simulink model "Disturbed_H_PB"  (R2023a)
settings: Solver=VariableStepAuto  StartTime=0.0  StopTime=ttot  RelTol=1e-3
InitFcn:
  | run("Trajectory_Planning_Francesco.m");
  | 
  | % Defining important terms
  | 
  | g=9.81;
  | A=[zeros(3) eye(3);zeros(3) zeros(3)];
  | B=[zeros(3);eye(3)];
  | 
  | % Computing gain PD+
  | 
  | Ke_He=[diag([10 10 10]),diag([10 10 10])];
  | Kp_He=[diag([100 100 100]),diag([1 1 10])];
  | 
  | Kp_PB=[100*diag([1 1 1]),diag([0.5 0.5 10])];
values from neighbouring files (symbols this model uses):
  Ib = diag([1.2416 1.2416 2*1.2416])    [Trajectory_Planning_Francesco.m]
  K3 = flip(G3.Denominator{1})    [Trajectory_Planning_Francesco.m]
  lin_vel_0 = [dot_x0 dot_y0 dot_z0]    [Trajectory_Planning_Francesco.m]
  mass = 1.2    [Trajectory_Planning_Francesco.m]
  pos_0 = [Poses(1,1) Poses(1,2) Poses(1,3)]    [Trajectory_Planning_Francesco.m]
  Ts = 0.001    [Trajectory_Planning_Francesco.m]
undefined symbols (not defined in the file or in its folder): DiscIntNeverNeededParam
libraries: robotcorelib x2, uavutilslib x2
settings Model: Creator=fabioruggiero  LastModifiedBy=39388
settings ModelReferenceCC: EnableRefExpFcnMdlSchedulingChecks=on

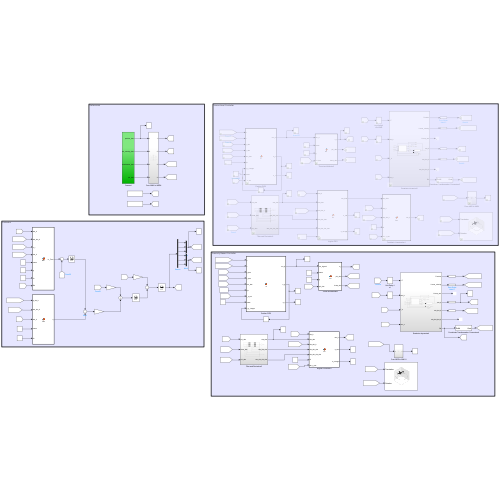
[thumbnail: Simulink's stored preview of the top-level diagram]
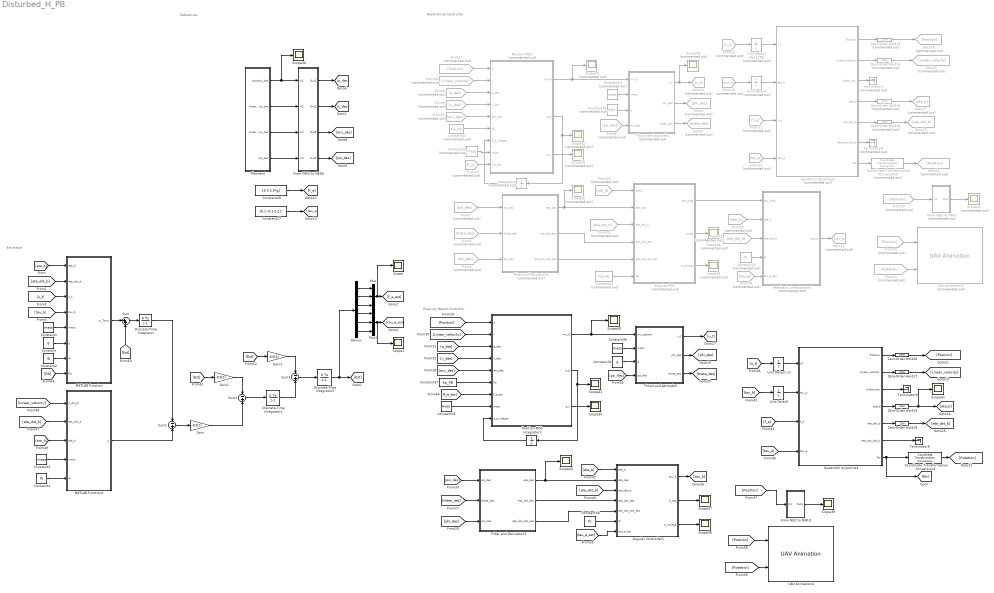
== system Disturbed_H_PB ==
  note: Estimator
  note: References
  note: Hierarchical Controller
  note: Passivity Based Controller
  Angular Controller1 : MATLAB Function  TreatAsAtomicUnit=on
  Angular PID1 : MATLAB Function  Commented=on  TreatAsAtomicUnit=on
  Constant : Constant  Value=g
  Constant{1,3,35..36} (4 alike) : Constant  Value=mass
  Constant18 : Constant  Commented=on  Value=9.81
  Constant19 : Constant  Commented=on  Value=Ib
  Constant2 : Constant  Value=Ib
  Constant20 : Constant  Commented=on  Value=mass
  Constant21 : Constant  Commented=on  Value=Kp_He
  Constant22 : Constant  Commented=on  Value=Ke_He
  Constant23 : Constant  Commented=on  Value=mass
  Constant27 : Constant  Value=[0.1 -0.1 0.2]'  SampleTime=Ts
  Constant28 : Constant  Value=[0 0 2.5*g]  SampleTime=Ts
  Constant34 : Constant  Value=g
  Constant37 : Constant  Value=Kp_PB
  Constant38 : Constant  Value=Ib
  Constant4 : Constant  Value=Ib
  Coordinate Transformation Conversion3 : robotcorelib/Coordinate Transformation Conversion  Commented=on  InputRepresentation=Rotation Matrix  InputEulerSequence=ZYX  ShowTrVecInputPort=on  OutputRepresentation=Quaternion  OutputEulerSequence=ZYX  ShowTrVecOutputPort=on  SimulateUsing=Interpreted execution
  Coordinate Transformation Conversion4 : robotcorelib/Coordinate Transformation Conversion  InputRepresentation=Rotation Matrix  InputEulerSequence=ZYX  ShowTrVecInputPort=on  OutputRepresentation=Quaternion  OutputEulerSequence=ZYX  ShowTrVecOutputPort=on  SimulateUsing=Interpreted execution
  Demux : Demux  Outputs=6
  Discrete-Time Integrator : DiscreteIntegrator  gainval=1  SampleTime=Ts  ICPrevOutput=DiscIntNeverNeededParam  ICPrevScaledInput=DiscIntNeverNeededParam
  Discrete-Time Integrator1 : DiscreteIntegrator  gainval=1  SampleTime=Ts  ICPrevOutput=DiscIntNeverNeededParam  ICPrevScaledInput=DiscIntNeverNeededParam
  Discrete-Time Integrator2 : DiscreteIntegrator  gainval=1  SampleTime=Ts  ICPrevOutput=DiscIntNeverNeededParam  ICPrevScaledInput=DiscIntNeverNeededParam
  Feedback Linearization1 : MATLAB Function  Commented=on  TreatAsAtomicUnit=on
  Filter and Derivation2 : Subsystem  Commented=on
  Filter and Derivation3 : Subsystem
  From NED to NWU : Subsystem  Commented=on
  From NED to NWU1 : Subsystem
  From NWU to NED6 : Subsystem
  From10 : From  Commented=on  GotoTag=acc_des
  From11 : From  Commented=on  GotoTag=f_e
  From12 : From  Commented=on  GotoTag=tau_e
  From13 : From  Commented=on  GotoTag=f_e
  From14 : From  Commented=on  GotoTag=tau_e
  From15 : From  Commented=on  GotoTag=u_t
  From16 : From  Commented=on  GotoTag=tau_b
  From17 : From  Commented=on  GotoTag=Position
  From18 : From  Commented=on  GotoTag=Linear_velocity
  From19 : From  Commented=on  GotoTag=Position
  From20 : From  Commented=on  GotoTag=Position
  From21 : From  Commented=on  GotoTag=Rotation
  From22 : From  Commented=on  GotoTag=eta_b
  From23 : From  Commented=on  GotoTag=eta_b
  From24 : From  Commented=on  GotoTag=eta_dot_b
  From25 : From  Commented=on  GotoTag=eta_dot_b
  From4 : From  Commented=on  GotoTag=phi_des
  From5 : From  Commented=on  GotoTag=theta_des
  From6 : From  Commented=on  GotoTag=psi_des
  From7 : From  Commented=on  GotoTag=psi_des
  From8 : From  Commented=on  GotoTag=p_des
  From9 : From  Commented=on  GotoTag=v_des
  Gain : Gain  Gain=K3(1)
  Gain1 : Gain  Gain=K3(2)
  Gain2 : Gain  Gain=K3(3)
  Goto12 : Goto  Commented=on  GotoTag=u_t
  Goto13 : Goto  Commented=on  GotoTag=tau_b
  Goto14 : Goto  Commented=on  GotoTag=Position
  Goto15 : Goto  Commented=on  GotoTag=Linear_velocity
  Goto16 : Goto  Commented=on  GotoTag=Rotation
  Goto17 : Goto  Commented=on  GotoTag=eta_b
  Goto18 : Goto  Commented=on  GotoTag=eta_dot_b
  Goto4 : Goto  Commented=on  GotoTag=phi_des
  Goto5 : Goto  Commented=on  GotoTag=theta_des
  Integrator2 : Integrator  Commented=on  InitialCondition=[0 0 0]'
  Integrator3 : Integrator  InitialCondition=[0 0 0]'
  MATLAB Function : MATLAB Function  TreatAsAtomicUnit=on
  MATLAB Function1 : MATLAB Function  TreatAsAtomicUnit=on
  Mux : Mux  Inputs=3
  Mux1 : Mux  Inputs=3
  Planner4 : Subsystem
  Position PID2 : MATLAB Function  Commented=on  TreatAsAtomicUnit=on
  Position PID3 : MATLAB Function  TreatAsAtomicUnit=on
  Quadrotor dynamics3 : Subsystem  Commented=on
  Quadrotor dynamics4 : Subsystem
  Scope{,1,30,36..43} (11 alike) : Scope
  Scope{24,28..29,31..35} (8 alike) : Scope  Commented=on
  Sum : Sum  Inputs=|++
  Sum1 : Sum  Inputs=-+
  Sum2 : Sum  Inputs=-+
  Sum3 : Sum  Inputs=-+
  Terminator6 : Terminator  Commented=on
  Terminator7 : Terminator  Commented=on
  Terminator8 : Terminator
  Terminator9 : Terminator
  Thrust and Attitude2 : MATLAB Function  Commented=on  TreatAsAtomicUnit=on
  Thrust and Attitude3 : MATLAB Function  TreatAsAtomicUnit=on
  UAV Animation3 : uavutilslib/UAV Animation  Commented=on  UAVType=Multirotor  UAVSize=1  InertialZDirection=Down  SampleTime=Ts
  UAV Animation4 : uavutilslib/UAV Animation  UAVType=Multirotor  UAVSize=1  InertialZDirection=Down  SampleTime=Ts
  Unit Delay1 u0=12N2 : UnitDelay  Commented=on  InitialCondition=11.77  SampleTime=Ts
  Unit Delay1 u1 : UnitDelay  InitialCondition=11.77  SampleTime=Ts
  Unit Delay4 : UnitDelay  Commented=on  InitialCondition=[0 0 0]'  SampleTime=Ts
  Unit Delay5 : UnitDelay  InitialCondition=[0 0 0]'  SampleTime=Ts
  Zero-Order Hold{13..16} (4 alike) : ZeroOrderHold  Commented=on  SampleTime=Ts
  Zero-Order Hold{17..20} (4 alike) : ZeroOrderHold  SampleTime=Ts
  wires:
  Angular PID1/3(e_omega) -> Scope29/1
  Constant21/1 -> Position PID2/6(Kp)
  From NED to NWU/1(Out1) -> Scope31/1
  Constant18/1 -> Thrust and Attitude2/3(g)
  Quadrotor dynamics3/3(Linear_acc) -> Terminator7/1
  Filter and Derivation2/3(eta_dot_dot_des) -> Angular PID1/5(eta_dot_dot_des)
  Constant19/1 -> Feedback Linearization1/4(Ib)
  Unit Delay4/1 -> Quadrotor dynamics3/2(tau_b)
  Position PID2/2(e_p) -> Scope32/1, Integrator2/1
  Unit Delay1 u0=12N2/1 -> Quadrotor dynamics3/1(uT)
  Position PID2/1(mu_d) -> Scope33/1, Thrust and Attitude2/1(mu_d)
  Quadrotor dynamics3/7(Rb) -> Coordinate Transformation Conversion3/1
  Thrust and Attitude2/3(theta_des) -> Goto5/1
  Angular PID1/2(e_eta) -> Scope28/1
  Constant22/1 -> Angular PID1/6(Ke)
  Zero-Order Hold13/1 -> Goto14/1
  Constant20/1 -> Thrust and Attitude2/2(mass)
  From5/1 -> Filter and Derivation2/2(theta_des)
  Quadrotor dynamics3/6(eta_dot_dot_b) -> Terminator6/1
  Thrust and Attitude2/1(u_t) -> Scope34/1, Goto12/1
  Quadrotor dynamics3/2(Linear_velocity) -> Zero-Order Hold14/1
  From4/1 -> Filter and Derivation2/3(phi_des)
  Quadrotor dynamics3/4(eta_b) -> Zero-Order Hold16/1
  Filter and Derivation2/2(eta_dot_des) -> Angular PID1/4(eta_dot_des)
  Quadrotor dynamics3/5(eta_dot_b) -> Zero-Order Hold15/1
  Thrust and Attitude2/2(phi_des) -> Goto4/1
  Angular PID1/1(tau_tilde) -> Feedback Linearization1/1(tau_tilde)
  Position PID2/3(e_v) -> Scope24/1
  Quadrotor dynamics3/1(Position) -> Zero-Order Hold13/1
  Integrator2/1 -> Position PID2/7(e_p_integer)
  Planner4/3(linear_acceleration_des) -> From NWU to NED6/3(In3)
  Planner4/1(position_des) -> Scope36/1, From NWU to NED6/1(In1)
  Planner4/2(linear_velocity_des) -> From NWU to NED6/2(In2)
  Planner4/4(psi_des) -> From NWU to NED6/4(In4)
  From NWU to NED6/1(Out1) -> [p_des]
  From NWU to NED6/2(Out2) -> [v_des]
  From NWU to NED6/3(Out3) -> [acc_des]
  From NWU to NED6/4(Out4) -> [psi_des]
  From6/1 -> Thrust and Attitude2/4(psi_des)
  From7/1 -> Filter and Derivation2/1(psi_des)
  From8/1 -> Position PID2/3(p_des)
  From9/1 -> Position PID2/4(v_des)
  From10/1 -> Position PID2/5(acc_des)
  Constant27/1 -> [tau_e]
  Constant28/1 -> [f_e]
  From11/1 -> Quadrotor dynamics3/3(f_e)
  From12/1 -> Quadrotor dynamics3/4(tau_e)
  From13/1 -> Position PID2/9(f_e_est)
  From14/1 -> Feedback Linearization1/5(tau_e_est)
  From15/1 -> Unit Delay1 u0=12N2/1
  Feedback Linearization1/1(tau_b) -> Goto13/1
  From16/1 -> Unit Delay4/1
  From17/1 -> Position PID2/1(p)
  Zero-Order Hold14/1 -> Goto15/1
  From18/1 -> Position PID2/2(v)
  Constant23/1 -> Position PID2/8(mass)
  From19/1 -> From NED to NWU/1(In1)
  From20/1 -> UAV Animation3/1
  Coordinate Transformation Conversion3/1 -> Goto16/1
  From21/1 -> UAV Animation3/2
  Zero-Order Hold16/1 -> Goto17/1
  From22/1 -> Angular PID1/1(eta_b)
  From23/1 -> Feedback Linearization1/2(eta_b)
  Zero-Order Hold15/1 -> Goto18/1
  From24/1 -> Feedback Linearization1/3(eta_dot_b)
  From25/1 -> Angular PID1/3(eta_dot_b)
  Filter and Derivation2/1(eta_des) -> Scope35/1, Angular PID1/2(eta_des)
  Thrust and Attitude3/2(phi_des) -> [phi_des]
  Filter and Derivation3/2(eta_dot_des) -> Angular Controller1/4(eta_dot_des)
  [f_e] -> Quadrotor dynamics4/3(f_e)
  Angular Controller1/2(e_eta) -> Scope37/1
  Constant36/1 -> Thrust and Attitude3/2(mass)
  Quadrotor dynamics4/5(eta_dot_b) -> Zero-Order Hold18/1
  Quadrotor dynamics4/1(Position) -> Zero-Order Hold20/1
  Zero-Order Hold20/1 -> [Position]
  Filter and Derivation3/3(eta_dot_dot_des) -> Angular Controller1/5(eta_dot_dot_des)
  Constant35/1 -> Position PID3/8(mass)
  Thrust and Attitude3/3(theta_des) -> [theta_des]
  Unit Delay1 u1/1 -> Quadrotor dynamics4/1(uT)
  Filter and Derivation3/1(eta_des) -> Angular Controller1/2(eta_des), Scope43/1
  [theta_des] -> Filter and Derivation3/2(theta_des)
  Angular Controller1/3(e_omega) -> Scope38/1
  Constant38/1 -> Angular Controller1/6(Ib)
  Position PID3/2(e_p) -> Integrator3/1, Scope41/1
  [phi_des] -> Filter and Derivation3/3(phi_des)
  Constant34/1 -> Thrust and Attitude3/3(g)
  Zero-Order Hold19/1 -> [eta_b], Scope42/1
  Unit Delay5/1 -> Quadrotor dynamics4/2(tau_b)
  Position PID3/3(e_v) -> Scope30/1
  Quadrotor dynamics4/2(Linear_velocity) -> Zero-Order Hold17/1
  Quadrotor dynamics4/4(eta_b) -> Zero-Order Hold19/1
  Quadrotor dynamics4/7(Rb) -> [Rb], Coordinate Transformation Conversion4/1
  Quadrotor dynamics4/3(Linear_acc) -> Terminator9/1
  [tau_e] -> Quadrotor dynamics4/4(tau_e)
  Constant37/1 -> Position PID3/6(Kp)
  Integrator3/1 -> Position PID3/9(e_p_integer)
  Quadrotor dynamics4/6(eta_dot_dot_b) -> Terminator8/1
  [Position] -> Position PID3/1(p)
  [Linear_velocity] -> Position PID3/2(v)
  [p_des] -> Position PID3/3(p_des)
  [v_des] -> Position PID3/4(v_des)
  [acc_des] -> Position PID3/5(acc_des)
  [psi_des] -> Filter and Derivation3/1(psi_des)
  [psi_des] -> Thrust and Attitude3/4(psi_des)
  [f_e_est] -> Position PID3/7(f_e_est)
  Position PID3/1(mu_d) -> Scope40/1, Thrust and Attitude3/1(mu_signed)
  [u_t] -> Unit Delay1 u1/1
  [Rotation] -> UAV Animation4/2
  [Position] -> From NED to NWU1/1(In1)
  From NED to NWU1/1(Out1) -> Scope39/1
  [Position] -> UAV Animation4/1
  Coordinate Transformation Conversion4/1 -> [Rotation]
  Zero-Order Hold17/1 -> [Linear_velocity]
  Zero-Order Hold18/1 -> [eta_dot_b]
  [eta_dot_b] -> Angular Controller1/3(eta_dot_b)
  [eta_b] -> Angular Controller1/1(eta_b)
  Angular Controller1/1(tau_b) -> [tau_b]
  [tau_b] -> Unit Delay5/1
  [tau_e_est] -> Angular Controller1/7(tau_e_est)
  Thrust and Attitude3/1(u_t) -> [u_t]
  [eta_dot_b] -> MATLAB Function/2(eta_dot_b)
  [u_t] -> MATLAB Function/3(u_t)
  [tau_b] -> MATLAB Function/4(tau_b)
  [eta_b] -> MATLAB Function/1(eta_b)
  [Rb] -> MATLAB Function/8(Rb)
  Constant/1 -> MATLAB Function/6(g)
  Constant1/1 -> MATLAB Function/5(mass)
  Constant2/1 -> MATLAB Function/7(Ib)
  [eta_dot_b] -> MATLAB Function1/2(eta_dot_b)
  [Linear_velocity] -> MATLAB Function1/1(p_dot_b)
  [eta_b] -> MATLAB Function1/3(eta_b)
  Constant3/1 -> MATLAB Function1/4(mass)
  Constant4/1 -> MATLAB Function1/5(Ib)
  MATLAB Function/1(m_Term) -> Sum/1
  Sum/1 -> Discrete-Time Integrator/1
  [Est] -> Sum/2
  Discrete-Time Integrator/1 -> Sum1/1
  MATLAB Function1/1(q) -> Sum1/2
  Sum1/1 -> Gain/1
  Gain/1 -> Sum2/2
  [Est] -> Gain1/1
  Gain1/1 -> Sum2/1
  Sum2/1 -> Discrete-Time Integrator1/1
  [Est] -> Gain2/1
  Gain2/1 -> Sum3/1
  Discrete-Time Integrator1/1 -> Sum3/2
  Sum3/1 -> Discrete-Time Integrator2/1
  Discrete-Time Integrator2/1 -> Demux/1, [Est]
  Demux/1 -> Mux/1
  Demux/2 -> Mux/2
  Demux/3 -> Mux/3
  Demux/4 -> Mux1/1
  Demux/5 -> Mux1/2
  Demux/6 -> Mux1/3
  Mux/1 -> Scope/1, [f_e_est]
  Mux1/1 -> Scope1/1, [tau_e_est]

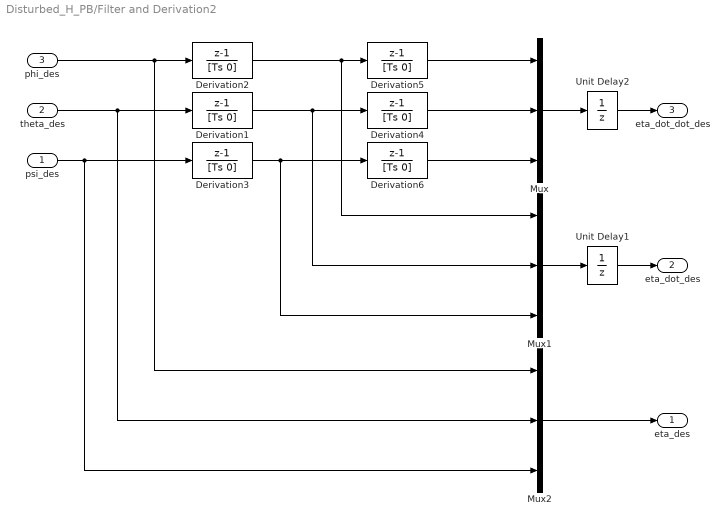
== system Disturbed_H_PB/Filter and Derivation2 ==
  psi_des : Inport
  theta_des : Inport  Port=2
  phi_des : Inport  Port=3
  Derivation{1..6} (6 alike) : DiscreteTransferFcn  Numerator=[1 -1]  Denominator=[Ts 0]  SampleTime=Ts
  Mux : Mux  Inputs=3
  Mux1 : Mux  Inputs=3
  Mux2 : Mux  Inputs=3
  Unit Delay1 : UnitDelay  InitialCondition=[0 0 0]  SampleTime=Ts
  Unit Delay2 : UnitDelay  InitialCondition=[0 0 0]  SampleTime=Ts
  eta_des : Outport
  eta_dot_des : Outport  Port=2
  eta_dot_dot_des : Outport  Port=3
  wires:
  theta_des/1 -> Derivation1/1, Mux2/2
  Derivation1/1 -> Derivation4/1, Mux1/2
  Derivation3/1 -> Derivation6/1, Mux1/3
  Derivation2/1 -> Derivation5/1, Mux1/1
  Derivation6/1 -> Mux/3
  phi_des/1 -> Derivation2/1, Mux2/1
  psi_des/1 -> Derivation3/1, Mux2/3
  Mux1/1 -> Unit Delay1/1
  Mux/1 -> Unit Delay2/1
  Mux2/1 -> eta_des/1
  Unit Delay1/1 -> eta_dot_des/1
  Unit Delay2/1 -> eta_dot_dot_des/1
  Derivation4/1 -> Mux/2
  Derivation5/1 -> Mux/1

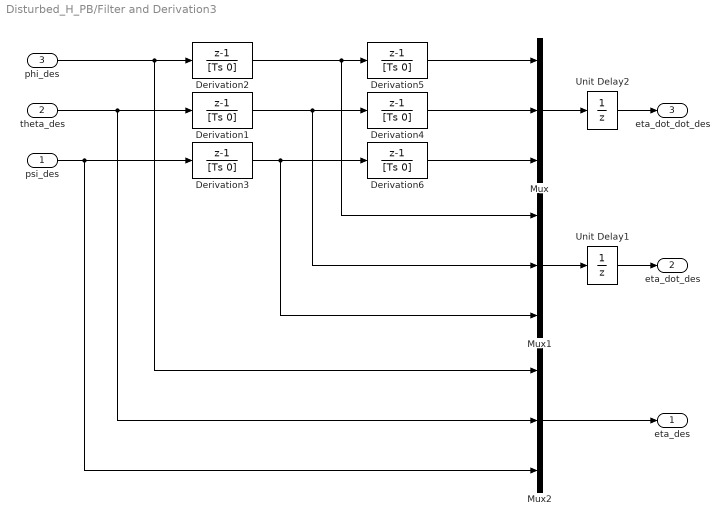
== system Disturbed_H_PB/Filter and Derivation3 ==
  psi_des : Inport
  theta_des : Inport  Port=2
  phi_des : Inport  Port=3
  Derivation{1..6} (6 alike) : DiscreteTransferFcn  Numerator=[1 -1]  Denominator=[Ts 0]  SampleTime=Ts
  Mux : Mux  Inputs=3
  Mux1 : Mux  Inputs=3
  Mux2 : Mux  Inputs=3
  Unit Delay1 : UnitDelay  InitialCondition=[0 0 0]  SampleTime=Ts
  Unit Delay2 : UnitDelay  InitialCondition=[0 0 0]  SampleTime=Ts
  eta_des : Outport
  eta_dot_des : Outport  Port=2
  eta_dot_dot_des : Outport  Port=3
  wires:
  theta_des/1 -> Derivation1/1, Mux2/2
  Derivation1/1 -> Derivation4/1, Mux1/2
  Derivation3/1 -> Derivation6/1, Mux1/3
  Derivation2/1 -> Derivation5/1, Mux1/1
  Derivation6/1 -> Mux/3
  phi_des/1 -> Derivation2/1, Mux2/1
  psi_des/1 -> Derivation3/1, Mux2/3
  Mux1/1 -> Unit Delay1/1
  Mux/1 -> Unit Delay2/1
  Mux2/1 -> eta_des/1
  Unit Delay1/1 -> eta_dot_des/1
  Unit Delay2/1 -> eta_dot_dot_des/1
  Derivation4/1 -> Mux/2
  Derivation5/1 -> Mux/1

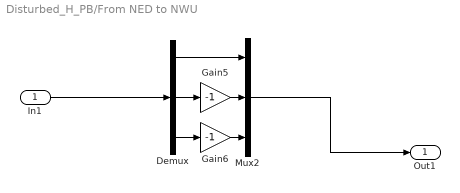
== system Disturbed_H_PB/From NED to NWU ==
  In1 : Inport
  Demux : Demux  Outputs=3
  Gain5 : Gain  Gain=-1
  Gain6 : Gain  Gain=-1
  Mux2 : Mux  Inputs=3
  Out1 : Outport
  wires:
  Gain5/1 -> Mux2/2
  In1/1 -> Demux/1
  Gain6/1 -> Mux2/3
  Demux/3 -> Gain6/1
  Mux2/1 -> Out1/1
  Demux/1 -> Mux2/1
  Demux/2 -> Gain5/1

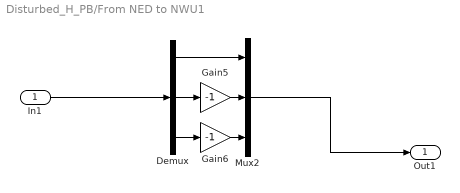
== system Disturbed_H_PB/From NED to NWU1 ==
  In1 : Inport
  Demux : Demux  Outputs=3
  Gain5 : Gain  Gain=-1
  Gain6 : Gain  Gain=-1
  Mux2 : Mux  Inputs=3
  Out1 : Outport
  wires:
  Gain5/1 -> Mux2/2
  In1/1 -> Demux/1
  Gain6/1 -> Mux2/3
  Demux/3 -> Gain6/1
  Mux2/1 -> Out1/1
  Demux/1 -> Mux2/1
  Demux/2 -> Gain5/1

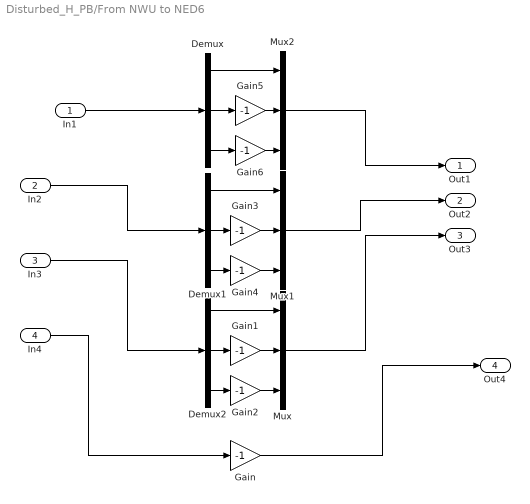
== system Disturbed_H_PB/From NWU to NED6 ==
  In1 : Inport
  In2 : Inport  Port=2
  In3 : Inport  Port=3
  In4 : Inport  Port=4
  Demux : Demux  Outputs=3
  Demux1 : Demux  Outputs=3
  Demux2 : Demux  Outputs=3
  Gain{,1..6} (7 alike) : Gain  Gain=-1
  Mux : Mux  Inputs=3
  Mux1 : Mux  Inputs=3
  Mux2 : Mux  Inputs=3
  Out1 : Outport
  Out2 : Outport  Port=2
  Out3 : Outport  Port=3
  Out4 : Outport  Port=4
  wires:
  Gain5/1 -> Mux2/2
  Gain3/1 -> Mux1/2
  In1/1 -> Demux/1
  Gain6/1 -> Mux2/3
  Demux2/2 -> Gain1/1
  Mux/1 -> Out3/1
  Gain4/1 -> Mux1/3
  Demux/3 -> Gain6/1
  Demux1/1 -> Mux1/1
  Mux2/1 -> Out1/1
  Demux1/3 -> Gain4/1
  Demux1/2 -> Gain3/1
  Gain1/1 -> Mux/2
  Demux/1 -> Mux2/1
  In3/1 -> Demux2/1
  Demux/2 -> Gain5/1
  Demux2/1 -> Mux/1
  Gain2/1 -> Mux/3
  Demux2/3 -> Gain2/1
  In2/1 -> Demux1/1
  Mux1/1 -> Out2/1
  Gain/1 -> Out4/1
  In4/1 -> Gain/1

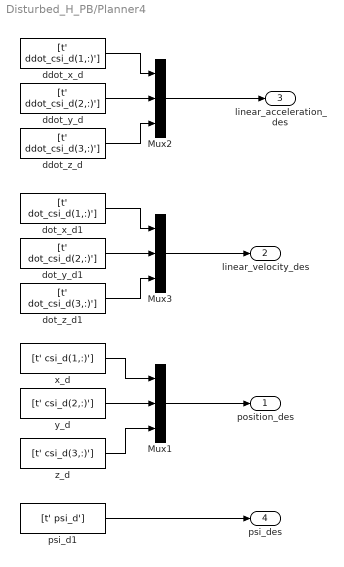
== system Disturbed_H_PB/Planner4 ==
  Mux1 : Mux  Inputs=3
  Mux2 : Mux  Inputs=3
  Mux3 : Mux  Inputs=3
  ddot_x_d : FromWorkspace  VariableName=[t' ddot_csi_d(1,:)']  SampleTime=Ts
  ddot_y_d : FromWorkspace  VariableName=[t' ddot_csi_d(2,:)']  SampleTime=Ts
  ddot_z_d : FromWorkspace  VariableName=[t' ddot_csi_d(3,:)']  SampleTime=Ts
  dot_x_d1 : FromWorkspace  VariableName=[t' dot_csi_d(1,:)']  SampleTime=Ts
  dot_y_d1 : FromWorkspace  VariableName=[t' dot_csi_d(2,:)']  SampleTime=Ts
  dot_z_d1 : FromWorkspace  VariableName=[t' dot_csi_d(3,:)']  SampleTime=Ts
  psi_d1 : FromWorkspace  VariableName=[t' psi_d']  SampleTime=Ts
  x_d : FromWorkspace  VariableName=[t' csi_d(1,:)']  SampleTime=Ts
  y_d : FromWorkspace  VariableName=[t' csi_d(2,:)']  SampleTime=Ts
  z_d : FromWorkspace  VariableName=[t' csi_d(3,:)']  SampleTime=Ts
  position_des : Outport
  linear_velocity_des : Outport  Port=2
  linear_acceleration_des : Outport  Port=3
  psi_des : Outport  Port=4
  wires:
  y_d/1 -> Mux1/2
  z_d/1 -> Mux1/3
  x_d/1 -> Mux1/1
  ddot_y_d/1 -> Mux2/2
  ddot_z_d/1 -> Mux2/3
  ddot_x_d/1 -> Mux2/1
  Mux2/1 -> linear_acceleration_des/1
  Mux1/1 -> position_des/1
  dot_y_d1/1 -> Mux3/2
  dot_z_d1/1 -> Mux3/3
  dot_x_d1/1 -> Mux3/1
  Mux3/1 -> linear_velocity_des/1
  psi_d1/1 -> psi_des/1

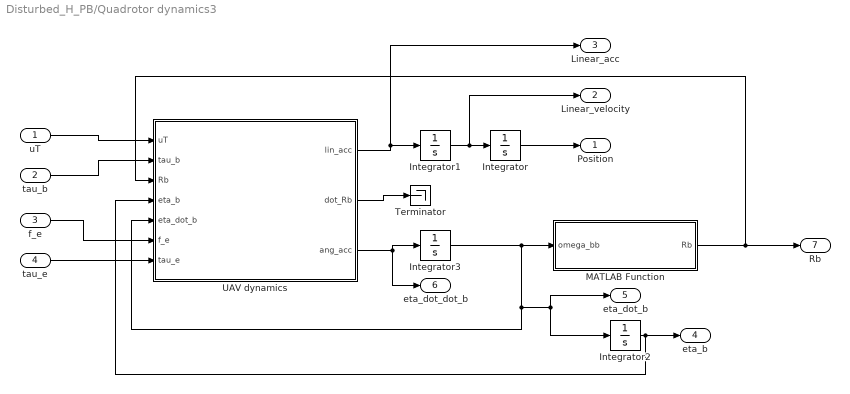
== system Disturbed_H_PB/Quadrotor dynamics3 ==
  uT : Inport
  tau_b : Inport  Port=2
  f_e : Inport  Port=3
  tau_e : Inport  Port=4
  Integrator : Integrator  InitialCondition=-pos_0
  Integrator1 : Integrator  InitialCondition=lin_vel_0
  Integrator2 : Integrator  InitialCondition=[0 0 0]
  Integrator3 : Integrator  InitialCondition=[0 0 0]
  MATLAB Function : MATLAB Function  TreatAsAtomicUnit=on
  Terminator : Terminator
  UAV dynamics : MATLAB Function  TreatAsAtomicUnit=on
  Position : Outport
  Linear_velocity : Outport  Port=2
  Linear_acc : Outport  Port=3
  eta_b : Outport  Port=4
  eta_dot_b : Outport  Port=5
  eta_dot_dot_b : Outport  Port=6
  Rb : Outport  Port=7
  wires:
  tau_b/1 -> UAV dynamics/2(tau_b)
  Integrator/1 -> Position/1
  UAV dynamics/3(ang_acc) -> Integrator3/1, eta_dot_dot_b/1
  UAV dynamics/1(lin_acc) -> Linear_acc/1, Integrator1/1
  uT/1 -> UAV dynamics/1(uT)
  Integrator1/1 -> Linear_velocity/1, Integrator/1
  Integrator3/1 -> UAV dynamics/5(eta_dot_b), eta_dot_b/1, Integrator2/1, MATLAB Function/1(omega_bb)
  UAV dynamics/2(dot_Rb) -> Terminator/1
  MATLAB Function/1(Rb) -> Rb/1, UAV dynamics/3(Rb)
  Integrator2/1 -> UAV dynamics/4(eta_b), eta_b/1
  f_e/1 -> UAV dynamics/6(f_e)
  tau_e/1 -> UAV dynamics/7(tau_e)

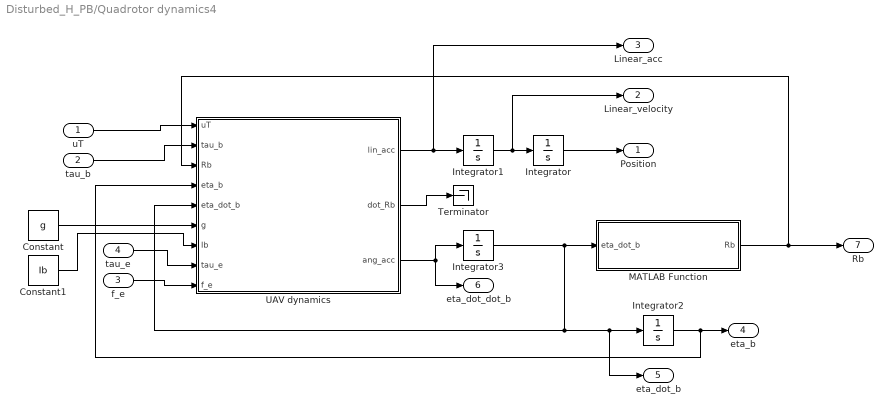
== system Disturbed_H_PB/Quadrotor dynamics4 ==
  uT : Inport
  tau_b : Inport  Port=2
  f_e : Inport  Port=3
  tau_e : Inport  Port=4
  Constant : Constant  Value=g
  Constant1 : Constant  Value=Ib
  Integrator : Integrator  InitialCondition=-pos_0
  Integrator1 : Integrator  InitialCondition=lin_vel_0
  Integrator2 : Integrator  InitialCondition=[0 0 0]
  Integrator3 : Integrator  InitialCondition=[0 0 0]
  MATLAB Function : MATLAB Function  TreatAsAtomicUnit=on
  Terminator : Terminator
  UAV dynamics : MATLAB Function  TreatAsAtomicUnit=on
  Position : Outport
  Linear_velocity : Outport  Port=2
  Linear_acc : Outport  Port=3
  eta_b : Outport  Port=4
  eta_dot_b : Outport  Port=5
  eta_dot_dot_b : Outport  Port=6
  Rb : Outport  Port=7
  wires:
  tau_b/1 -> UAV dynamics/2(tau_b)
  Integrator/1 -> Position/1
  UAV dynamics/3(ang_acc) -> Integrator3/1, eta_dot_dot_b/1
  UAV dynamics/1(lin_acc) -> Linear_acc/1, Integrator1/1
  uT/1 -> UAV dynamics/1(uT)
  Integrator1/1 -> Linear_velocity/1, Integrator/1
  Integrator3/1 -> eta_dot_b/1, Integrator2/1, UAV dynamics/5(eta_dot_b), MATLAB Function/1(eta_dot_b)
  UAV dynamics/2(dot_Rb) -> Terminator/1
  MATLAB Function/1(Rb) -> Rb/1, UAV dynamics/3(Rb)
  Integrator2/1 -> UAV dynamics/4(eta_b), eta_b/1
  f_e/1 -> UAV dynamics/9(f_e)
  tau_e/1 -> UAV dynamics/8(tau_e)
  Constant/1 -> UAV dynamics/6(g)
  Constant1/1 -> UAV dynamics/7(Ib)

== matlab function Disturbed_H_PB/Thrust and Attitude2 ==
  data: mu_d input; mass input; g input; u_t output; psi_des input; phi_des output; theta_des output
function [u_t, phi_des, theta_des] = fcn(mu_d, mass, g, psi_des)

u_t=mass*sqrt(mu_d(1)^(2)+mu_d(2)^(2)+(mu_d(3)-g)^(2));
phi_des=asin(mass/u_t*(mu_d(2)*cos(psi_des)-mu_d(1)*sin(psi_des)));
theta_des=atan((mu_d(1)*cos(psi_des)+mu_d(2)*sin(psi_des))/(mu_d(3)-g));

end

== matlab function Disturbed_H_PB/Angular Controller1 ==
  data: eta_b input; eta_des input; eta_dot_b input; tau_b output; eta_dot_des input; eta_dot_dot_des input; e_eta output; e_omega output; Ib input; tau_e_est input
function [tau_b, e_eta, e_omega] = fcn(eta_b, eta_des, eta_dot_b, eta_dot_des, eta_dot_dot_des, Ib, tau_e_est)

e_eta = eta_b-eta_des;
e_omega = eta_dot_b-eta_dot_des;

Do=eye(3);
sigma=20;
v=20;
Ko=sigma*Do;

eta_r_dot=eta_dot_des-sigma*e_eta;
eta_r_dot_dot=eta_dot_dot_des-v*e_omega;
v_eta=e_omega+sigma*e_eta;

phi=eta_b(1);
theta=eta_b(2);
psi=eta_b(3);
phi_dot=eta_dot_b(1);
theta_dot=eta_dot_b(2);
psi_dot=eta_dot_b(3);

%definition trasformation matrix
Q=[1 ,     0      , -sin(theta);
   0 , cos(phi)   ,  cos(theta)*sin(phi);
   0 ,-sin(phi)   ,  cos(theta)*cos(phi)];

Q_dot=[0 ,     0            , -cos(theta)*theta_dot            ;
       0 , -sin(phi)*phi_dot,  cos(phi)*phi_dot*cos(theta)-sin(phi)*sin(theta)*theta_dot;
       0 , -cos(phi)*phi_dot, -sin(phi)*phi_dot*cos(theta)-cos(phi)*theta_dot*sin(theta)];

S=skew(Q*eta_dot_b);

C=Q'*S*Ib*Q+Q'*Ib*Q_dot;
M=Q'*Ib*Q;

tau_b=Q'\(M*eta_r_dot_dot+C*eta_r_dot-tau_e_est-Do*v_eta-Ko*e_eta);

%skew symmetric operator
function S = skew(v)
if(numel(v)~= 1)
S= [0 -v(3) v(2); 
    v(3) 0 -v(1);
    -v(2) v(1) 0];
else
S= zeros(3);
end

== matlab function Disturbed_H_PB/Position PID3 ==
  data: p input; v input; p_des input; mu_d output; v_des input; acc_des input; e_p output; e_v output; Kp input; f_e_est input; mass input; e_p_integer input
function [mu_d, e_p, e_v] = fcn(p, v, p_des, v_des, acc_des, Kp, f_e_est, mass, e_p_integer)

g=9.81;
e_p=p-p_des;
e_v=v-v_des;
e=[e_p;e_v];
Ki=2.5*diag([100 100 100]);

mu_d = -Kp*e - Ki*e_p_integer + acc_des - f_e_est/mass;

if mu_d(3)>g
    mu_d(3)=9.8;
end

end

== matlab function Disturbed_H_PB/Quadrotor dynamics4/MATLAB Function ==
  data: eta_dot_b input; Rb output
function Rb = fcn(eta_dot_b)

Rb = expm(skew(eta_dot_b));
end

function S = skew(v)
if(numel(v)~= 1)
S= [0 -v(3) v(2); 
    v(3) 0 -v(1);
    -v(2) v(1) 0];
else
S= zeros(3);
end
end

== matlab function Disturbed_H_PB/Quadrotor dynamics4/UAV dynamics ==
  data: uT input size=1; tau_b input size=3; lin_acc output size=3; Rb input size=[3,3]; eta_b input; eta_dot_b input size=3; dot_Rb output size=[3,3]; ang_acc output size=3; mass parameter size=1; g input; Ib input; tau_e input; f_e input
function [lin_acc, dot_Rb, ang_acc] = fcn(uT, tau_b, Rb, eta_b, eta_dot_b, mass, g, Ib, tau_e, f_e)

phi=eta_b(1);
theta=eta_b(2);
phi_dot=eta_dot_b(1);
theta_dot=eta_dot_b(2);

Q=[1 ,     0      , -sin(theta);
   0 , cos(phi)   ,  cos(theta)*sin(phi);
   0 ,-sin(phi)   ,  cos(theta)*cos(phi)];

Q_dot=[0 ,     0            , -cos(theta)*theta_dot            ;
       0 , -sin(phi)*phi_dot,  cos(phi)*phi_dot*cos(theta)-sin(phi)*sin(theta)*theta_dot;
       0 , -cos(phi)*phi_dot, -sin(phi)*phi_dot*cos(theta)-cos(phi)*theta_dot*sin(theta)];

S=skew(Q*eta_dot_b);

C=Q'*S*Ib*Q+Q'*Ib*Q_dot;
M=Q'*Ib*Q;

lin_acc = g*[0 0 1]'-(uT/mass)*Rb*[0 0 1]' + f_e/mass;
dot_Rb = Rb*skew(eta_dot_b);
ang_acc = M\(-C*eta_dot_b + Q'*tau_b + tau_e);

end

function S = skew(v)
if(numel(v)~= 1)
S= [0 -v(3) v(2); 
    v(3) 0 -v(1);
    -v(2) v(1) 0];
else
S= zeros(3);
end
end

== matlab function Disturbed_H_PB/Thrust and Attitude3 ==
  data: mu_signed input; mass input; g input; u_t output; psi_des input; phi_des output; theta_des output
function [u_t, phi_des, theta_des] = fcn(mu_signed, mass, g, psi_des)

u_t=mass*sqrt(mu_signed(1)^(2)+mu_signed(2)^(2)+(mu_signed(3)-g)^(2));
phi_des=asin(mass/u_t*(mu_signed(2)*cos(psi_des)-mu_signed(1)*sin(psi_des)));
theta_des=atan((mu_signed(1)*cos(psi_des)+mu_signed(2)*sin(psi_des))/(mu_signed(3)-g));

end

== matlab function Disturbed_H_PB/MATLAB Function1 ==
  data: p_dot_b input; q output; eta_dot_b input; eta_b input; mass input; Ib input
function q = fcn(p_dot_b, eta_dot_b, eta_b, mass, Ib)

phi=eta_b(1);
theta=eta_b(2);

Q=[1 ,     0      , -sin(theta);
   0 , cos(phi)   ,  cos(theta)*sin(phi);
   0 ,-sin(phi)   ,  cos(theta)*cos(phi)];

M=Q'*Ib*Q;

q = [mass*eye(3) zeros(3); zeros(3) M]*[p_dot_b;eta_dot_b];

== matlab function Disturbed_H_PB/MATLAB Function ==
  data: eta_b input; m_Term output; eta_dot_b input; u_t input; tau_b input; mass input; g input; Ib input; Rb input
function m_Term = fcn(eta_b, eta_dot_b, u_t, tau_b, mass, g, Ib, Rb)

phi=eta_b(1);
theta=eta_b(2);
phi_dot=eta_dot_b(1);
theta_dot=eta_dot_b(2);

Q=[1 ,     0      , -sin(theta);
   0 , cos(phi)   ,  cos(theta)*sin(phi);
   0 ,-sin(phi)   ,  cos(theta)*cos(phi)];

Q_dot=[0 ,     0            , -cos(theta)*theta_dot            ;
       0 , -sin(phi)*phi_dot,  cos(phi)*phi_dot*cos(theta)-sin(phi)*sin(theta)*theta_dot;
       0 , -cos(phi)*phi_dot, -sin(phi)*phi_dot*cos(theta)-cos(phi)*theta_dot*sin(theta)];

S=skew(Q*eta_dot_b);

C=Q'*S*Ib*Q+Q'*Ib*Q_dot;

m_Term = [mass*g*[0 0 1]'-u_t*Rb*[0 0 1]'; C'*eta_dot_b+Q'*tau_b] ;

end

function S = skew(v)
if(numel(v)~= 1)
S= [0 -v(3) v(2); 
    v(3) 0 -v(1);
    -v(2) v(1) 0];
else
S= zeros(3);
end
end

== matlab function Disturbed_H_PB/Angular PID1 ==
  data: eta_b input; eta_des input; eta_dot_b input; tau_tilde output; eta_dot_des input; eta_dot_dot_des input; e_eta output; e_omega output; Ke input
function [tau_tilde, e_eta, e_omega] = fcn(eta_b, eta_des, eta_dot_b, eta_dot_des, eta_dot_dot_des, Ke)

e_eta = eta_b-eta_des;
e_omega = eta_dot_b-eta_dot_des;
e=[e_eta;e_omega];

tau_tilde = -Ke*e + eta_dot_dot_des;
end

== matlab function Disturbed_H_PB/Feedback Linearization1 ==
  data: tau_tilde input; tau_b output; eta_b input; eta_dot_b input; Ib input; tau_e_est input
function tau_b = fcn(tau_tilde,eta_b,eta_dot_b, Ib,tau_e_est)

%inizialization
phi=eta_b(1);
theta=eta_b(2);
psi=eta_b(3);
phi_dot=eta_dot_b(1);
theta_dot=eta_dot_b(2);
psi_dot=eta_dot_b(3);

%definition trasformation matrix
Q=[1 ,     0      , -sin(theta);
   0 , cos(phi)   ,  cos(theta)*sin(phi);
   0 ,-sin(phi)   ,  cos(theta)*cos(phi)];

Q_dot=[0 ,     0            , -cos(theta)*theta_dot            ;
       0 , -sin(phi)*phi_dot,  cos(phi)*phi_dot*cos(theta)-sin(phi)*sin(theta)*theta_dot;
       0 , -cos(phi)*phi_dot, -sin(phi)*phi_dot*cos(theta)-cos(phi)*theta_dot*sin(theta)];

S=skew(Q*eta_dot_b);

C=Q'*S*Ib*Q+Q'*Ib*Q_dot;
tau_b  = Ib*Q*tau_tilde + inv(Q')*C*eta_dot_b - Q'\tau_e_est;

%skew symmetric operator
function S = skew(v)
if(numel(v)~= 1)
S= [0 -v(3) v(2); 
    v(3) 0 -v(1);
    -v(2) v(1) 0];
else
S= zeros(3);
end

== matlab function Disturbed_H_PB/Position PID2 ==
  data: p input; v input; p_des input; mu_d output; v_des input; acc_des input; e_p output; e_v output; Kp input; e_p_integer input; mass input; f_e_est input
function [mu_d, e_p, e_v] = fcn(p, v, p_des, v_des, acc_des,Kp, e_p_integer, mass, f_e_est)

g=9.81;
e_p=p-p_des;
e_v=v-v_des;
e=[e_p;e_v];
Ki=2.5*diag([100 100 100]);


mu_d = -Kp*e -Ki*e_p_integer + acc_des-1/mass*f_e_est;


if(mu_d(3)>g)
    mu_d(3)=9.8;
end
end

== matlab function Disturbed_H_PB/Quadrotor dynamics3/MATLAB Function ==
  data: omega_bb input; Rb output
function Rb = fcn(omega_bb)

Rb = expm(skew(omega_bb));
end

function S = skew(v)
if(numel(v)~= 1)
S= [0 -v(3) v(2); 
    v(3) 0 -v(1);
    -v(2) v(1) 0];
else
S= zeros(3);
end
end

== matlab function Disturbed_H_PB/Quadrotor dynamics3/UAV dynamics ==
  data: uT input size=1; tau_b input size=3; lin_acc output size=3; Rb input size=[3,3]; eta_b input; eta_dot_b input size=3; dot_Rb output size=[3,3]; ang_acc output size=3; mass parameter size=1; Ib parameter size=[3,3]; f_e input; tau_e input
function [lin_acc, dot_Rb, ang_acc] = fcn(uT,tau_b,Rb,eta_b, eta_dot_b,mass, Ib, f_e, tau_e)

phi=eta_b(1);
theta=eta_b(2);
phi_dot=eta_dot_b(1);
theta_dot=eta_dot_b(2);

Q=[1 ,     0      , -sin(theta);
   0 , cos(phi)   ,  cos(theta)*sin(phi);
   0 ,-sin(phi)   ,  cos(theta)*cos(phi)];

Q_dot=[0 ,     0            , -cos(theta)*theta_dot            ;
       0 , -sin(phi)*phi_dot,  cos(phi)*phi_dot*cos(theta)-sin(phi)*sin(theta)*theta_dot;
       0 , -cos(phi)*phi_dot, -sin(phi)*phi_dot*cos(theta)-cos(phi)*theta_dot*sin(theta)];

S=skew(Q*eta_dot_b);

C=Q'*S*Ib*Q+Q'*Ib*Q_dot;
M=Q'*Ib*Q;

lin_acc = 9.81*[0 0 1]'-(uT/mass)*Rb*[0 0 1]'+1/mass*f_e;
dot_Rb = Rb*skew(eta_dot_b);
ang_acc = M\(-C*eta_dot_b + Q'*tau_b + tau_e);

end

function S = skew(v)
if(numel(v)~= 1)
S= [0 -v(3) v(2); 
    v(3) 0 -v(1);
    -v(2) v(1) 0];
else
S= zeros(3);
end
end
